simulink model "Helicopter_Simulink_Model"  (R2015a)
settings: Solver=ode45  StartTime=0.0  StopTime=80  RelTol=1e-3
values from neighbouring files (symbols this model uses):
  C_0 = [[C(1,:)] ... (first row only)    [setup_lab_heli_3d_skeleton.m]
  K = lqr(A, B, Qx, Qu)    [setup_lab_heli_3d_skeleton.m]
  K_r = (-C_0*inv(A - B*K)*B)^-1    [setup_lab_heli_3d_skeleton.m]
  L_mod = place(A',C',P_L_model)'    [setup_lab_heli_3d_skeleton.m]
undefined symbols (not defined in the file or in its folder): A, B, C, D
libraries: simulink x4
settings Model: Creator=Owner  LastModifiedBy=Owner
settings HardwareCC: TargetLongLongMode=on  TargetIntDivRoundTo=Zero  TargetEndianess=LittleEndian  TargetHWDeviceType=MATLAB Host  ProdEqTarget=off
settings RTWCC: SystemTargetFile=rsim.tlc  TemplateMakefile=rsim_default_tmf  Description=Rapid Simulation Target
settings RSimTargetCC: ERTMultiwordTypeDef=System defined  ERTMultiwordLength=256

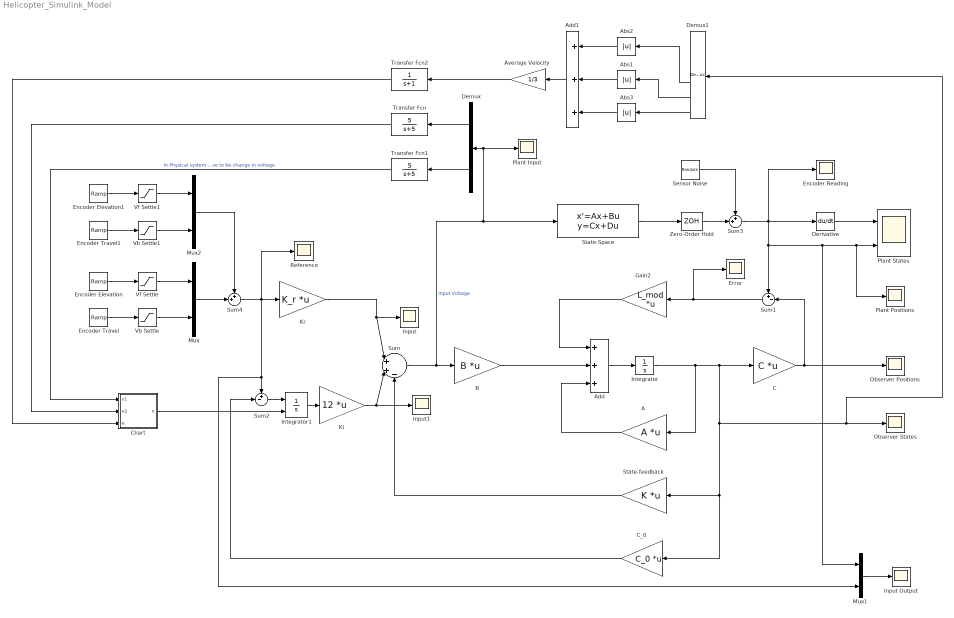
== system Helicopter_Simulink_Model ==
  A : Gain  Gain=A  Multiplication=Matrix(K*u)
  Abs1 : Abs
  Abs2 : Abs
  Abs3 : Abs
  Add : Sum  Inputs=+++
  Add1 : Sum  Inputs=+++
  Average Velocity : Gain  Gain=1/3
  B : Gain  Gain=B  Multiplication=Matrix(K*u)
  C : Gain  Gain=C  Multiplication=Matrix(K*u)
  C_0 : Gain  Gain=C_0  Multiplication=Matrix(K*u)
  Chart : Stateflow chart  TreatAsAtomicUnit=on
  Demux : Demux  Outputs=2
  Demux1 : Demux  Outputs=6
  Derivative : Derivative
  Encoder Elevation : simulink/Sources/Ramp  slope=-0.125  start=30  X0=0.4995
  Encoder Elevation1 : simulink/Sources/Ramp  slope=0.125  start=0  X0=0
  Encoder Reading : Scope
      settings: SaveName=ScopeData6
  Encoder Travel : simulink/Sources/Ramp  slope=0  start=0  X0=0
  Encoder Travel1 : simulink/Sources/Ramp  slope=0  start=0  X0=0
  Error : Scope
      settings: SaveName=ScopeData3
  Gain2 : Gain  Gain=L_mod  Multiplication=Matrix(K*u)
  Input : Scope
  Input Output : Scope
      settings: SaveName=ScopeData7
  Input1 : Scope
      settings: SaveName=ScopeData11
  Integrator : Integrator
  Integrator1 : Integrator  ExternalReset=rising
  Ki : Gain  Gain=12  Multiplication=Matrix(K*u)
  Kr : Gain  Gain=K_r  Multiplication=Matrix(K*u)
  Mux : Mux  Inputs=2
  Mux1 : Mux  Inputs=2
  Mux2 : Mux  Inputs=2
  Observer Positions : Scope
      settings: SaveName=ScopeData4
  Observer States : Scope
      settings: SaveName=ScopeData2
  Plant Input : Scope
      settings: SaveName=ScopeData9
  Plant Positions : Scope
      settings: SaveName=ScopeData5
  Plant States : Scope  NumInputPorts=2
      settings: YMin=-5~-5  YMax=5~5
  Reference : Scope
      settings: SaveName=ScopeData8
  Sensor Noise : UniformRandomNumber  Minimum=-0.0002  Maximum=0.0002  SampleTime=0.012
  State-Space : StateSpace  A=A  B=B  C=C  D=D  X0=0
  State-feedback : Gain  Gain=K  Multiplication=Matrix(K*u)
  Sum : Sum  Inputs=|++-
  Sum1 : Sum  Inputs=+-|
  Sum2 : Sum  Inputs=+-|
  Sum3 : Sum  Inputs=++|
  Sum4 : Sum  Inputs=++|
  Transfer Fcn : TransferFcn  Numerator=[5]  Denominator=[1 5]
  Transfer Fcn1 : TransferFcn  Numerator=[5]  Denominator=[1 5]
  Transfer Fcn2 : TransferFcn  Denominator=[1 1]
  Vb Settle : Saturate  UpperLimit=0.4995  LowerLimit=-1
  Vb Settle1 : Saturate  UpperLimit=0.4995  LowerLimit=-1
  Vf Settle : Saturate  UpperLimit=0  LowerLimit=-0.4995
  Vf Settle1 : Saturate  UpperLimit=0.4995  LowerLimit=-1
  Zero-Order Hold : ZeroOrderHold  SampleTime=0.012
  wires:
  Encoder Elevation/1 -> Vf Settle/1
  Encoder Travel/1 -> Vb Settle/1
  Vf Settle/1 -> Mux/1
  Vb Settle/1 -> Mux/2
  Sum/1 -> Plant Input/1, Demux/1, State-Space/1, B/1  "Input Voltage"
  B/1 -> Add/2
  A/1 -> Add/3
  Add/1 -> Integrator/1
  Integrator/1 -> C/1, Demux1/1, Observer States/1, C_0/1, State-feedback/1, A/1
  Sum3/1 -> Encoder Reading/1, Derivative/1, Sum1/1, Mux1/1, Plant Positions/1, Plant States/2
  Gain2/1 -> Add/1
  Derivative/1 -> Plant States/1
  State-feedback/1 -> Sum/3
  Sum4/1 -> Mux1/2, Sum2/1, Reference/1, Kr/1
  Kr/1 -> Sum/1, Input/1
  Sum2/1 -> Integrator1/1
  C_0/1 -> Sum2/2
  Ki/1 -> Sum/2, Input1/1
  Integrator1/1 -> Ki/1
  Sum1/1 -> Error/1, Gain2/1
  Sensor Noise/1 -> Sum3/1
  State-Space/1 -> Zero-Order Hold/1
  Zero-Order Hold/1 -> Sum3/2
  Mux1/1 -> Input Output/1
  Encoder Elevation1/1 -> Vf Settle1/1
  Encoder Travel1/1 -> Vb Settle1/1
  Vf Settle1/1 -> Mux2/1
  Vb Settle1/1 -> Mux2/2
  Mux2/1 -> Sum4/1
  Mux/1 -> Sum4/2
  Demux/1 -> Transfer Fcn/1
  Demux/2 -> Transfer Fcn1/1
  Transfer Fcn/1 -> Chart/2(v2)
  Transfer Fcn1/1 -> Chart/1(v1)  "In Physical system this will have to be change in voltage"
  Chart/1(x) -> Integrator1/2
  Add1/1 -> Average Velocity/1
  Average Velocity/1 -> Transfer Fcn2/1
  C/1 -> Observer Positions/1, Sum1/2
  Demux1/4 -> Abs2/1
  Demux1/5 -> Abs1/1
  Demux1/6 -> Abs3/1
  Abs2/1 -> Add1/1
  Abs1/1 -> Add1/2
  Abs3/1 -> Add1/3
  Transfer Fcn2/1 -> Chart/3(e)

== stateflow chart Helicopter_Simulink_Model/Chart ==
  state Reset
    entry:
    x=0;
  state No_Reset
    entry:
    x=1;
  No_Reset -> Reset : [ (abs(v1) < 0.1) & (abs(v2) < 0.1) & (abs(e) < 0.002)]
  (default) -> No_Reset
  Reset -> No_Reset : [(abs(v1) > 0.1) | (abs(v2) > 0.1)| (abs(e) > 0.002)]
  data: v1 input; v2 input; x output; e input
